simulink model "NL_2DOF"  (R2019b)
settings: Solver=VariableStepAuto  StartTime=0.0  StopTime=200  RelTol=1e-3
InitFcn:
  | load("parameters.mat");
  | load("Coefficients.mat");
undefined symbols (not defined in the file): Dm, Dt, F_limit_pitch, g, Jp, Jy, k_pitch, k_py, k_yaw, k_yp, Mb, w_neg_0, w_neg_1, w_pos_0, w_pos_1
settings Model: Creator=laptop  LastModifiedBy=lbend

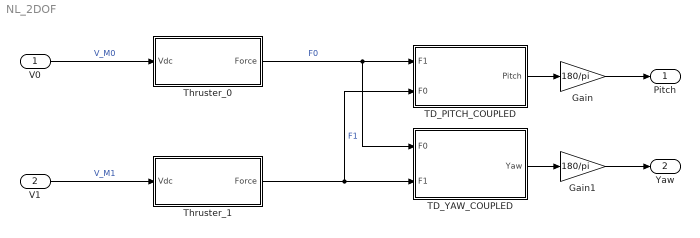
== system NL_2DOF ==
  V0 : Inport
  V1 : Inport  Port=2
  Gain : Gain  Gain=180/pi
  Gain1 : Gain  Gain=180/pi
  TD_PITCH_COUPLED : Subsystem
  TD_YAW_COUPLED : Subsystem
  Thruster_0 : Subsystem
  "Thruster_1 " : Subsystem
  Pitch : Outport
  Yaw : Outport  Port=2
  wires:
  V1/1 -> "Thruster_1 "/1(Vdc)  "V_M1"
  "Thruster_1 "/1(Force) -> TD_PITCH_COUPLED/2(F0), TD_YAW_COUPLED/2(F1)  "F1"
  V0/1 -> Thruster_0/1(Vdc)  "V_M0"
  Thruster_0/1(Force) -> TD_YAW_COUPLED/1(F0), TD_PITCH_COUPLED/1("F1 ")  "F0"
  TD_PITCH_COUPLED/1(Pitch) -> Gain/1
  Gain/1 -> Pitch/1
  TD_YAW_COUPLED/1("Yaw ") -> Gain1/1
  Gain1/1 -> Yaw/1

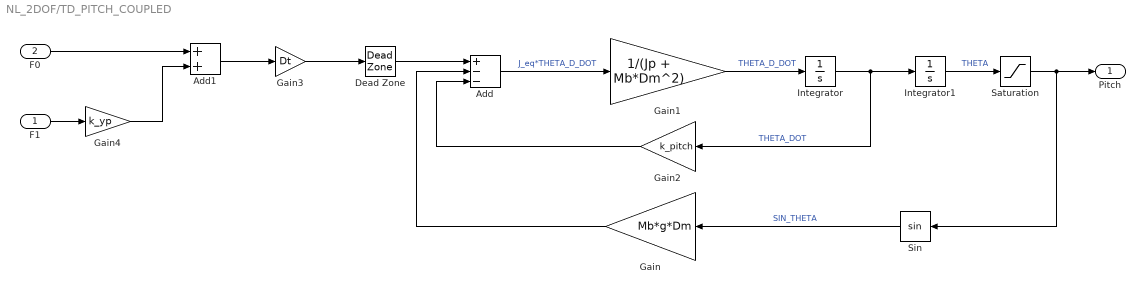
== system NL_2DOF/TD_PITCH_COUPLED ==
  "F1 " : Inport
  F0 : Inport  Port=2
  Add : Sum  Inputs=+--
  Add1 : Sum
  Dead Zone : DeadZone  LowerValue=F_limit_pitch/2  UpperValue=F_limit_pitch/2  SaturateOnIntegerOverflow=on
  Gain : Gain  Gain=Mb*g*Dm
  Gain1 : Gain  Gain=1/(Jp + Mb*Dm^2)
  Gain2 : Gain  Gain=k_pitch
  Gain3 : Gain  Gain=Dt
  Gain4 : Gain  Gain=k_yp
  Integrator : Integrator
  Integrator1 : Integrator
  Saturation : Saturate  UpperLimit=0.93  LowerLimit=-0.93
  Sin : Trigonometry
  Pitch : Outport
  wires:
  Gain2/1 -> Add/3
  Saturation/1 -> Sin/1, Pitch/1
  Sin/1 -> Gain/1  "SIN_THETA"
  Integrator/1 -> Integrator1/1, Gain2/1  "THETA_DOT"
  Add/1 -> Gain1/1  "J_eq*THETA_D_DOT"
  Gain1/1 -> Integrator/1  "THETA_D_DOT"
  Gain/1 -> Add/2
  Integrator1/1 -> Saturation/1  "THETA"
  Gain3/1 -> Dead Zone/1
  Dead Zone/1 -> Add/1
  Add1/1 -> Gain3/1
  F0/1 -> Add1/1
  "F1 "/1 -> Gain4/1
  Gain4/1 -> Add1/2

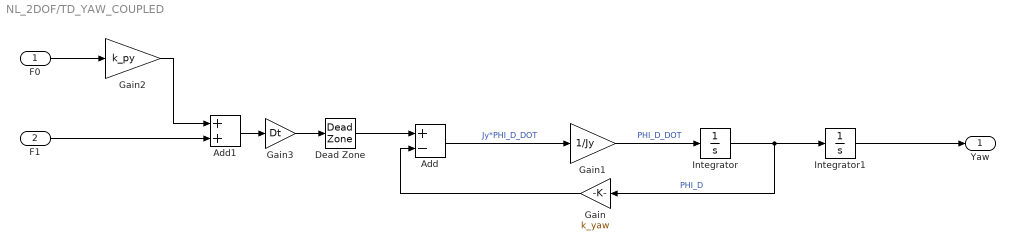
== system NL_2DOF/TD_YAW_COUPLED ==
  F0 : Inport
  F1 : Inport  Port=2
  Add : Sum  Inputs=+-
  Add1 : Sum
  Dead Zone : DeadZone  LowerValue=F_limit_yaw  UpperValue=F_limit_yaw  SaturateOnIntegerOverflow=on
  Gain : Gain  Gain=k_yaw
  Gain1 : Gain  Gain=1/Jy
  Gain2 : Gain  Gain=k_py
  Gain3 : Gain  Gain=Dt
  Integrator : Integrator
  Integrator1 : Integrator
  "Yaw " : Outport
  wires:
  Gain2/1 -> Add1/1
  Integrator/1 -> Integrator1/1, Gain/1  "PHI_D"
  Add1/1 -> Gain3/1
  Gain/1 -> Add/2
  Gain3/1 -> Dead Zone/1
  Add/1 -> Gain1/1  "Jy*PHI_D_DOT"
  Dead Zone/1 -> Add/1
  Gain1/1 -> Integrator/1  "PHI_D_DOT"
  F1/1 -> Add1/2
  F0/1 -> Gain2/1
  Integrator1/1 -> "Yaw "/1

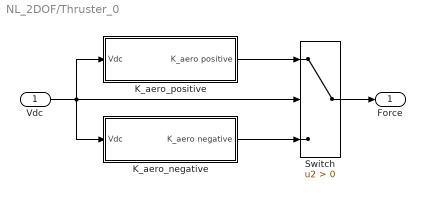
== system NL_2DOF/Thruster_0 ==
  Vdc : Inport
  K_aero_negative : Subsystem
  K_aero_positive : Subsystem
  Switch : Switch  Criteria=u2 > Threshold
  Force : Outport
  wires:
  Switch/1 -> Force/1
  K_aero_positive/1(K_aero positive) -> Switch/1
  Vdc/1 -> K_aero_positive/1(Vdc), K_aero_negative/1(Vdc), Switch/2
  K_aero_negative/1(K_aero negative) -> Switch/3

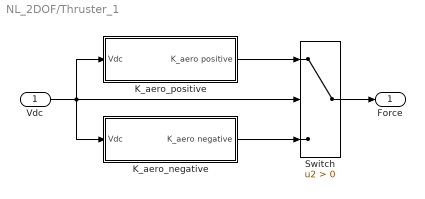
== system NL_2DOF/Thruster_1  ==
  Vdc : Inport
  K_aero_negative : Subsystem
  K_aero_positive : Subsystem
  Switch : Switch  Criteria=u2 > Threshold
  Force : Outport
  wires:
  Switch/1 -> Force/1
  K_aero_positive/1(K_aero positive) -> Switch/1
  Vdc/1 -> K_aero_negative/1(Vdc), Switch/2, K_aero_positive/1(Vdc)
  K_aero_negative/1(K_aero negative) -> Switch/3

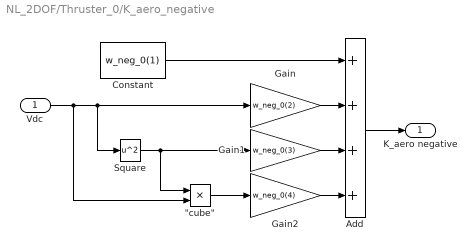
== system NL_2DOF/Thruster_0/K_aero_negative ==
  Vdc : Inport
  "\"cube\"" : Product  Inputs=**
  Add : Sum  Inputs=++++
  Constant : Constant  Value=w_neg_0(1)  SampleTime=0
  Gain : Gain  Gain=w_neg_0(2)
  Gain1 : Gain  Gain=w_neg_0(3)
  Gain2 : Gain  Gain=w_neg_0(4)
  Square : Math  Operator=square  SignedPower=off  SaturateOnIntegerOverflow=on
  K_aero negative : Outport
  wires:
  Constant/1 -> Add/1
  Vdc/1 -> "\"cube\""/2, Square/1, Gain/1
  Add/1 -> K_aero negative/1
  Gain/1 -> Add/2
  Square/1 -> "\"cube\""/1, Gain1/1
  Gain1/1 -> Add/3
  Gain2/1 -> Add/4
  "\"cube\""/1 -> Gain2/1

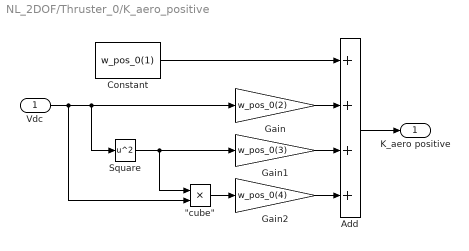
== system NL_2DOF/Thruster_0/K_aero_positive ==
  Vdc : Inport
  "\"cube\"" : Product  Inputs=**
  Add : Sum  Inputs=++++
  Constant : Constant  Value=w_pos_0(1)  SampleTime=0
  Gain : Gain  Gain=w_pos_0(2)
  Gain1 : Gain  Gain=w_pos_0(3)
  Gain2 : Gain  Gain=w_pos_0(4)
  Square : Math  Operator=square  SignedPower=off  SaturateOnIntegerOverflow=on
  K_aero positive : Outport
  wires:
  Constant/1 -> Add/1
  Vdc/1 -> Gain/1, Square/1, "\"cube\""/2
  Add/1 -> K_aero positive/1
  Gain/1 -> Add/2
  Square/1 -> "\"cube\""/1, Gain1/1
  Gain1/1 -> Add/3
  "\"cube\""/1 -> Gain2/1
  Gain2/1 -> Add/4

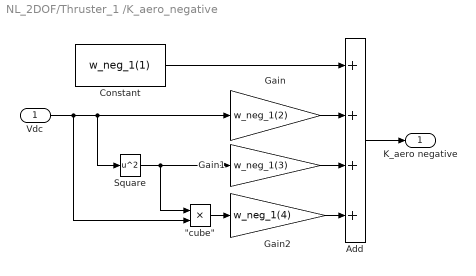
== system NL_2DOF/Thruster_1 /K_aero_negative ==
  Vdc : Inport
  "\"cube\"" : Product  Inputs=**
  Add : Sum  Inputs=++++
  Constant : Constant  Value=w_neg_1(1)  SampleTime=0
  Gain : Gain  Gain=w_neg_1(2)
  Gain1 : Gain  Gain=w_neg_1(3)
  Gain2 : Gain  Gain=w_neg_1(4)
  Square : Math  Operator=square  SignedPower=off  SaturateOnIntegerOverflow=on
  K_aero negative : Outport
  wires:
  Constant/1 -> Add/1
  Vdc/1 -> "\"cube\""/2, Square/1, Gain/1
  Add/1 -> K_aero negative/1
  Gain/1 -> Add/2
  Square/1 -> "\"cube\""/1, Gain1/1
  Gain1/1 -> Add/3
  Gain2/1 -> Add/4
  "\"cube\""/1 -> Gain2/1

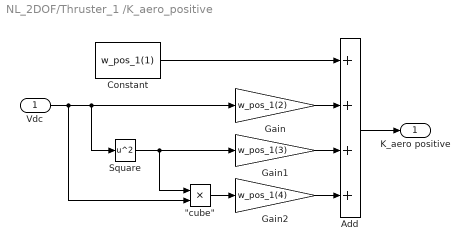
== system NL_2DOF/Thruster_1 /K_aero_positive ==
  Vdc : Inport
  "\"cube\"" : Product  Inputs=**
  Add : Sum  Inputs=++++
  Constant : Constant  Value=w_pos_1(1)  SampleTime=0
  Gain : Gain  Gain=w_pos_1(2)
  Gain1 : Gain  Gain=w_pos_1(3)
  Gain2 : Gain  Gain=w_pos_1(4)
  Square : Math  Operator=square  SignedPower=off  SaturateOnIntegerOverflow=on
  K_aero positive : Outport
  wires:
  Constant/1 -> Add/1
  Vdc/1 -> Gain/1, Square/1, "\"cube\""/2
  Add/1 -> K_aero positive/1
  Gain/1 -> Add/2
  Square/1 -> "\"cube\""/1, Gain1/1
  Gain1/1 -> Add/3
  "\"cube\""/1 -> Gain2/1
  Gain2/1 -> Add/4
